simulink model "Assignment_5"  (R2020b)
settings: Solver=VariableStepAuto  StartTime=0.0  StopTime=10.0  RelTol=1e-3
settings Model: Creator=Shantam Garg  LastModifiedBy=Shantam Garg

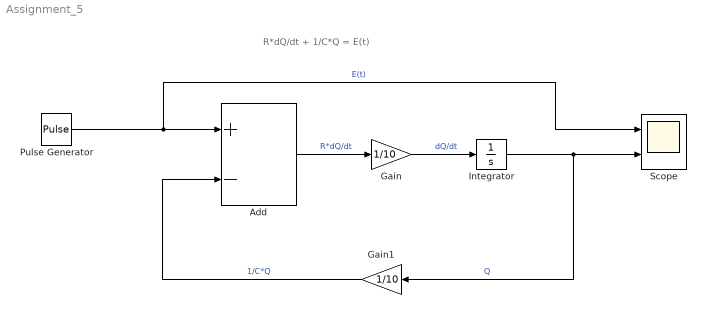
== system Assignment_5 ==
  note: R*dQ/dt + 1/C*Q = E(t)
  Add : Sum  Inputs=+-
  Gain : Gain  Gain=1/10
  Gain1 : Gain  Gain=1/10
  Integrator : Integrator
  Pulse Generator : DiscretePulseGenerator  PulseType=Time based  Period=.5  PulseWidth=10
  Scope : Scope  NumInputPorts=2
  wires:
  Add/1 -> Gain/1  "R*dQ/dt"
  Gain/1 -> Integrator/1  "dQ/dt"
  Integrator/1 -> Gain1/1, Scope/2  "Q"
  Gain1/1 -> Add/2  "1/C*Q"
  Pulse Generator/1 -> Add/1, Scope/1  "E(t)"
